simulink model "Engine_Model"  (R2025b)
settings: Solver=VariableStepAuto  StartTime=0.0  StopTime=10.0  RelTol=1e-3
settings Model: Creator=samue  LastModifiedBy=samue

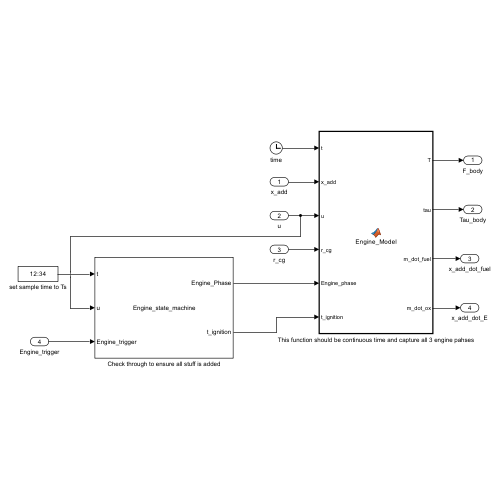
[thumbnail: Simulink's stored preview of the top-level diagram]
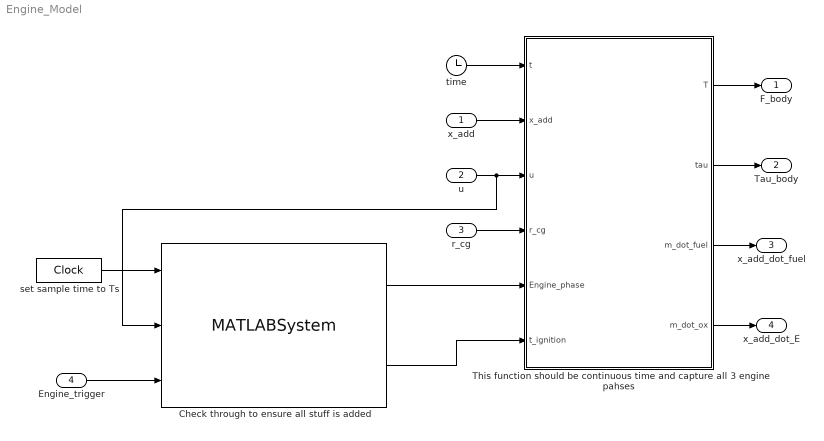
== system Engine_Model ==
  x_add : Inport
  u : Inport  Port=2
  r_cg : Inport  Port=3
  Engine_trigger : Inport  Port=4
  Check through to ensure all stuff is added : MATLABSystem  System=Engine_state_machine  SimulateUsing=Code generation
      mask Type: Engine_state_machine
  This function should be continuous time and capture all 3 engine pahses : MATLAB Function  TreatAsAtomicUnit=on
  set sample time to Ts : DigitalClock
  time : Clock
  F_body : Outport
  Tau_body : Outport  Port=2
  x_add_dot_fuel : Outport  Port=3
  x_add_dot_E : Outport  Port=4
  wires:
  x_add/1 -> This function should be continuous time and capture all 3 engine pahses/2(x_add)
  u/1 -> Check through to ensure all stuff is added/2, This function should be continuous time and capture all 3 engine pahses/3(u)
  This function should be continuous time and capture all 3 engine pahses/4(m_dot_ox) -> x_add_dot_E/1
  This function should be continuous time and capture all 3 engine pahses/3(m_dot_fuel) -> x_add_dot_fuel/1
  This function should be continuous time and capture all 3 engine pahses/2(tau) -> Tau_body/1
  This function should be continuous time and capture all 3 engine pahses/1(T) -> F_body/1
  r_cg/1 -> This function should be continuous time and capture all 3 engine pahses/4(r_cg)
  Engine_trigger/1 -> Check through to ensure all stuff is added/3
  Check through to ensure all stuff is added/1 -> This function should be continuous time and capture all 3 engine pahses/5(Engine_phase)
  time/1 -> This function should be continuous time and capture all 3 engine pahses/1(t)
  Check through to ensure all stuff is added/2 -> This function should be continuous time and capture all 3 engine pahses/6(t_ignition)
  set sample time to Ts/1 -> Check through to ensure all stuff is added/1

== matlab function Engine_Model/This function should be continuous time and capture all 3 engine pahses ==
  data: t input; x_add input; u input; r_cg input; Engine_phase input; T output; tau output; m_dot_fuel output; m_dot_ox output; t_ignition input
function [T, tau, m_dot_fuel, m_dot_ox] = Engine_Model(t, x_add, u, r_cg, Engine_phase, t_ignition)
% 
end
